simulink model "3_Bridge_rectifier"  (R2014a)
settings: Solver=ode23tb  StartTime=0.0  StopTime=.06  RelTol=1e-6
libraries: powerlib x15
settings Model: Creator=CHANDRA BABU  LastModifiedBy=Divya M
settings SolverCC: ZeroCrossControl=DisableAll
settings DataIOCC: SignalLoggingSaveFormat=ModelDataLogs
settings OptimizationCC: ExpressionDepthLimit=2147483647
settings DebuggingCC: UnderspecifiedInitializationDetection=Classic  FcnCallInpInsideContextMsg=UseLocalSettings  StateNameClashWarn=warning
settings GRTTargetCC: CombineOutputUpdateFcns=off  GRTInterface=on

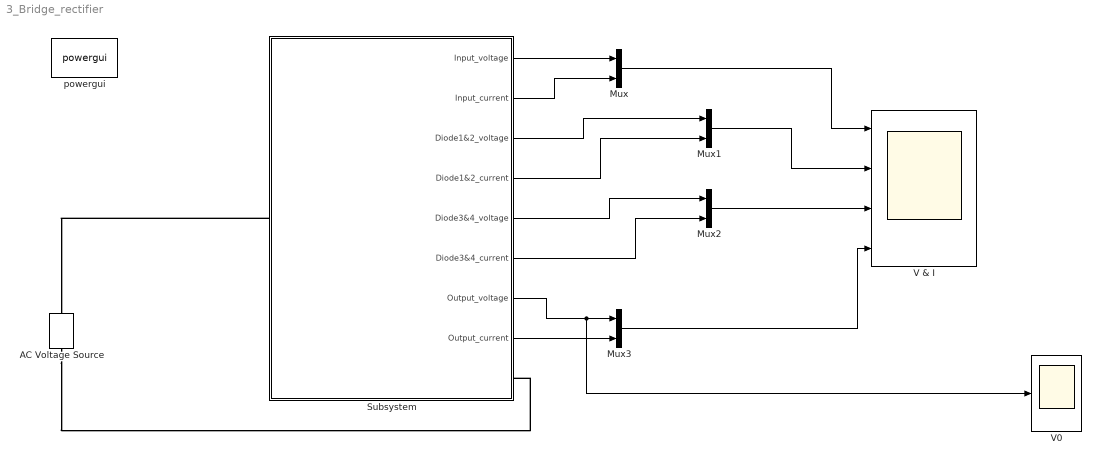
== system 3_Bridge_rectifier ==
  AC Voltage Source : powerlib/Electrical Sources/AC Voltage Source  Amplitude=5  Phase=0  Frequency=50  SampleTime=0  Measurements=None
  Mux{,1..3} (4 alike) : Mux  Inputs=2
  Subsystem : Subsystem
  V & I : Scope  NumInputPorts=4
      settings: YMin=-5~-5~-5~0  YMax=5~2~2~5
  V0 : Scope
      settings: SaveName=Outputvoltage
  powergui : powerlib/powergui  Priority=1  SimulationMode=Continuous  SolverType=Tustin  SampleTime=50e-6  frequency=60  SPID=off  DisableSnubberDevices=on  DisableRonSwitches=on  DisableVfSwitches=on  SwTol=0  Interpol=off  DisplayEquations=on  Ts=0  methode=off  frequencyindice=50  Pbase=100e6  ErrMax=1e-4  Iterations=50  UnitsV=kV  UnitsW=MW  FunctionMessages=off  echomessages=off  HookPort=off  EnableUseOfTLC=off  x0status=blocks  RestoreLinks=warning  ResistiveCurrentMeasurement=off  Frange=[0:2:500]  Ylog=off  Xlog=on  ShowGrid=off  save=off  variable=ZData  structure=Outputvoltage  ZoomFFT=on  StartTime=0.0  cycles=1  DisplayStyle=1  fundamental=50  FreqAxis=on  MaxFrequency=1000  frequencyindicesteady=1  RmsSteady=1  display=off
  wires:
  Mux/1 -> V & I/1
  Mux1/1 -> V & I/2
  Mux2/1 -> V & I/3
  Mux3/1 -> V & I/4
  Subsystem/1(Input_voltage) -> Mux/1
  Subsystem/2(Input_current) -> Mux/2
  Subsystem/3(Diode1&2_voltage) -> Mux1/1
  Subsystem/4(Diode1&2_current) -> Mux1/2
  Subsystem/5(Diode3&4_voltage) -> Mux2/1
  Subsystem/6(Diode3&4_current) -> Mux2/2
  Subsystem/7(Output_voltage) -> V0/1, Mux3/1
  Subsystem/8(Output_current) -> Mux3/2
  connections:
  Subsystem/LConn1 -- AC Voltage Source/RConn1
  AC Voltage Source/LConn1 -- Subsystem/RConn1

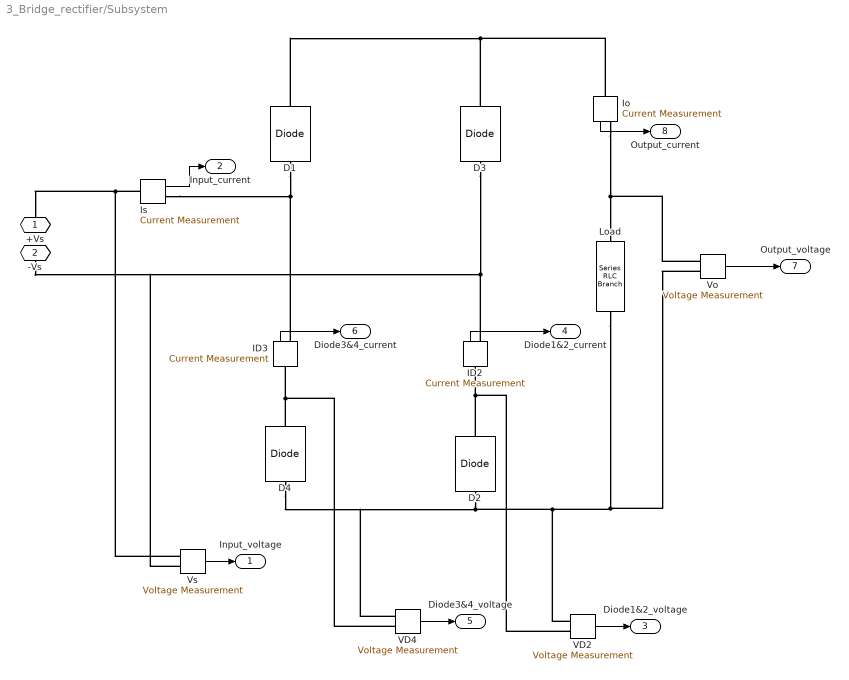
== system 3_Bridge_rectifier/Subsystem ==
  D{1..4} (4 alike) : powerlib/Power Electronics/Diode  Ron=0.001  Lon=0  Vf=0  IC=0  UseSnubber=off  Rs=500  Cs=250e-9  Measurements=off
  ID2 : powerlib/Measurements/Current Measurement  PhasorSimulation=off  OutputType=Complex  PSBequivalent=0
  ID3 : powerlib/Measurements/Current Measurement  PhasorSimulation=off  OutputType=Complex  PSBequivalent=0
  Io : powerlib/Measurements/Current Measurement  PhasorSimulation=off  OutputType=Complex  PSBequivalent=0
  Is : powerlib/Measurements/Current Measurement  PhasorSimulation=off  OutputType=Complex  PSBequivalent=0
  Load : powerlib/Elements/Series RLC Branch  LConnTagsString=__new0  RConnTagsString=__new0  BranchType=R  Resistance=2.5  Inductance=1e-3  SetiL0=off  InitialCurrent=0  Capacitance=1e-6  Setx0=off  InitialVoltage=0  Measurements=None
  VD2 : powerlib/Measurements/Voltage Measurement  PhasorSimulation=off  OutputType=Complex  PSBequivalent=0
  VD4 : powerlib/Measurements/Voltage Measurement  PhasorSimulation=off  OutputType=Complex  PSBequivalent=0
  Vo : powerlib/Measurements/Voltage Measurement  PhasorSimulation=off  OutputType=Complex  PSBequivalent=0
  Vs : powerlib/Measurements/Voltage Measurement  PhasorSimulation=off  OutputType=Complex  PSBequivalent=0
  +Vs : PMIOPort  Port=1  Side=Left
  -Vs : PMIOPort  Port=2  Side=Right
  Input_voltage : Outport
  Input_current : Outport  Port=2
  Diode1&2_voltage : Outport  Port=3
  Diode1&2_current : Outport  Port=4
  Diode3&4_voltage : Outport  Port=5
  Diode3&4_current : Outport  Port=6
  Output_voltage : Outport  Port=7
  Output_current : Outport  Port=8
  wires:
  Vo/1 -> Output_voltage/1
  Is/1 -> Input_current/1
  VD2/1 -> Diode1&2_voltage/1
  ID3/1 -> Diode3&4_current/1
  Io/1 -> Output_current/1
  VD4/1 -> Diode3&4_voltage/1
  Vs/1 -> Input_voltage/1
  ID2/1 -> Diode1&2_current/1
  connections:
  Is/RConn1 -- ID3/RConn1 -- D1/LConn1
  D4/RConn1 -- VD4/LConn2 -- ID3/LConn1
  D2/RConn1 -- VD2/LConn2 -- ID2/LConn1
  Is/LConn1 -- Vs/LConn1 -- +Vs/RConn1
  ID2/RConn1 -- Vs/LConn2 -- -Vs/RConn1 -- D3/LConn1
  Io/RConn1 -- Load/LConn1 -- Vo/LConn1
  Load/RConn1 -- Vo/LConn2 -- D4/LConn1 -- VD4/LConn1 -- D2/LConn1 -- VD2/LConn1
  Io/LConn1 -- D3/RConn1 -- D1/RConn1
